simulink model "FINAL_CHB_SPWM_FIXED_DC_5level2"  (R2014a)
settings: Solver=ode45  StartTime=0.0  StopTime=0.4  RelTol=1e-3
libraries: powerlib x22, simulink x4
settings Model: Creator=KOUSIK  LastModifiedBy=PRAKASH BABU

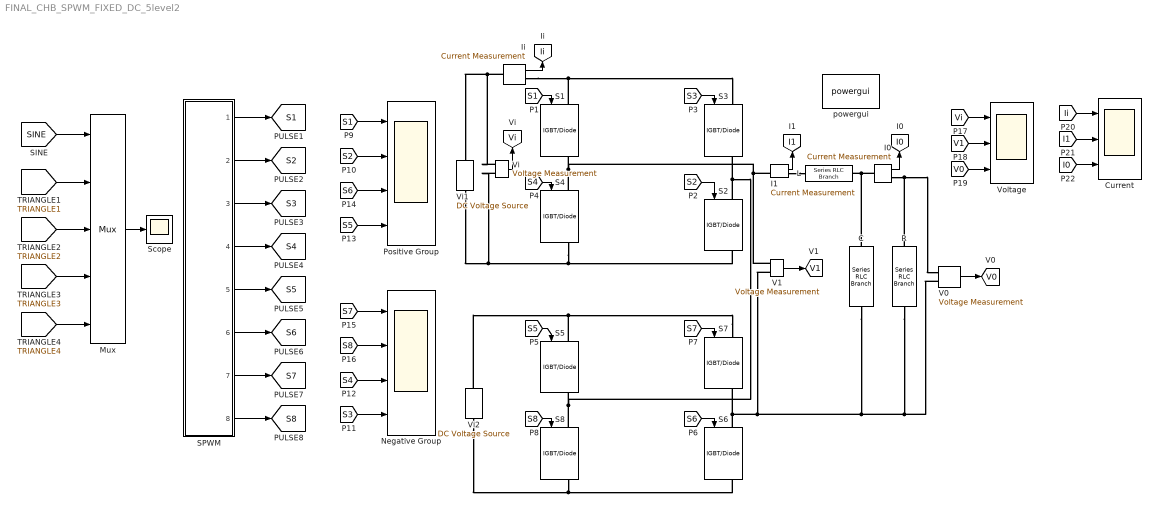
== system FINAL_CHB_SPWM_FIXED_DC_5level2 ==
  C : powerlib/Elements/Series RLC Branch  LConnTagsString=__new0  RConnTagsString=__new0  BranchType=C  Resistance=20  Inductance=5e-3  SetiL0=off  InitialCurrent=0  Capacitance=5.5e-6  Setx0=off  InitialVoltage=0  Measurements=None
  Current : Scope  NumInputPorts=3
      settings: TimeRange=0.1  YMin=-4~-4~-4  YMax=4~4~4  SaveName=current
  I0 : powerlib/Measurements/Current Measurement  PhasorSimulation=off  OutputType=Complex  PSBequivalent=0
  I1 : powerlib/Measurements/Current Measurement  PhasorSimulation=off  OutputType=Complex  PSBequivalent=0
  Ii : powerlib/Measurements/Current Measurement  PhasorSimulation=off  OutputType=Complex  PSBequivalent=0
  L : powerlib/Elements/Series RLC Branch  LConnTagsString=__new0  RConnTagsString=__new0  BranchType=L  Resistance=20  Inductance=35e-3  SetiL0=off  InitialCurrent=0  Capacitance=1e-6  Setx0=off  InitialVoltage=0  Measurements=None
  Mux : Mux  Inputs=5
  Negative Group : Scope  NumInputPorts=4
      settings: YMin=-5~-5~-5~-5  YMax=5~5~5~5  SaveName=negative
  Positive Group : Scope  NumInputPorts=4
      settings: YMin=-5~-5~-5~-5  YMax=5~5~5~5  SaveName=positive
  R : powerlib/Elements/Series RLC Branch  LConnTagsString=__new0  RConnTagsString=__new0  BranchType=R  Resistance=80  Inductance=5e-3  SetiL0=off  InitialCurrent=0  Capacitance=1e-6  Setx0=off  InitialVoltage=0  Measurements=None
  S{1..8} (8 alike) : powerlib/Power Electronics/IGBT//Diode  Ron=1e-3  Rs=1e5  Cs=inf  Measurements=on
  SPWM : Subsystem
  Scope : Scope
      settings: SaveName=sine
  V0 : powerlib/Measurements/Voltage Measurement  PhasorSimulation=off  OutputType=Complex  PSBequivalent=0
  "V1  " : powerlib/Measurements/Voltage Measurement  PhasorSimulation=off  OutputType=Complex  PSBequivalent=0
  Vi : powerlib/Measurements/Voltage Measurement  PhasorSimulation=off  OutputType=Complex  PSBequivalent=0
  Vi1 : powerlib/Electrical Sources/DC Voltage Source  Amplitude=115  Measurements=None
  Vi2 : powerlib/Electrical Sources/DC Voltage Source  Amplitude=115  Measurements=None
  Voltage : Scope  NumInputPorts=3
      settings: TimeRange=0.1  YMin=109~-300~-200  YMax=111~300~200  SaveName=voltage
  powergui : powerlib/powergui  Priority=1  SimulationMode=Discrete  SolverType=Tustin  SampleTime=50e-6  frequency=60  SPID=off  DisableSnubberDevices=off  DisableRonSwitches=off  DisableVfSwitches=off  SwTol=0  Interpol=off  DisplayEquations=off  Ts=0  methode=off  frequencyindice=0  Pbase=100e6  ErrMax=1e-4  Iterations=50  UnitsV=kV  UnitsW=MW  FunctionMessages=off  echomessages=off  HookPort=off  EnableUseOfTLC=off  x0status=blocks  RestoreLinks=warning  ResistiveCurrentMeasurement=off  Frange=[0:2:500]  Ylog=off  Xlog=on  ShowGrid=off  save=off  variable=ZData  structure=voltage  ZoomFFT=off  StartTime=0.02  cycles=1  DisplayStyle=1  fundamental=50  FreqAxis=off  MaxFrequency=1000  frequencyindicesteady=1  RmsSteady=1  display=off
  tag scope: I0=global, I1=global, Ii=global, S1=global, S2=global, S3=global, S4=global, S5=global, S6=global, S7=global, S8=global, V0=global, V1=global, Vi=global
  wires:
  [SINE] -> Mux/1
  [TRIANGLE1] -> Mux/2
  [TRIANGLE2] -> Mux/3
  [TRIANGLE3] -> Mux/4
  [TRIANGLE4] -> Mux/5
  Mux/1 -> Scope/1
  SPWM/1(1) -> [S1]
  SPWM/2(2) -> [S2]
  SPWM/4(4) -> [S4]
  SPWM/5(5) -> [S5]
  SPWM/6(6) -> [S6]
  SPWM/7(7) -> [S7]
  SPWM/8(8) -> [S8]
  SPWM/3(3) -> [S3]
  [S1] -> S1/1
  [S2] -> S2/1
  [S3] -> S3/1
  [S4] -> S4/1
  [S5] -> S5/1
  [S6] -> S6/1
  [S7] -> S7/1
  [S8] -> S8/1
  [S1] -> Positive Group/1
  [S2] -> Positive Group/2
  [S6] -> Positive Group/3
  [S5] -> Positive Group/4
  [S7] -> Negative Group/1
  [S8] -> Negative Group/2
  [S4] -> Negative Group/3
  [S3] -> Negative Group/4
  "V1  "/1 -> [V1]
  Ii/1 -> [Ii]
  Vi/1 -> [Vi]
  I1/1 -> [I1]
  V0/1 -> [V0]
  I0/1 -> [I0]
  [Vi] -> Voltage/1
  [V1] -> Voltage/2
  [V0] -> Voltage/3
  [Ii] -> Current/1
  [I1] -> Current/2
  [I0] -> Current/3
  connections:
  S1/LConn1 -- Ii/RConn1 -- S3/LConn1
  Vi1/LConn1 -- Vi/LConn2 -- S4/RConn1 -- S2/RConn1
  S4/LConn1 -- "V1  "/LConn1 -- I1/LConn1 -- S1/RConn1
  S7/LConn1 -- S5/LConn1 -- Vi2/RConn1
  Vi2/LConn1 -- S8/RConn1 -- S6/RConn1
  S3/RConn1 -- S2/LConn1 -- S8/LConn1 -- S5/RConn1
  S7/RConn1 -- "V1  "/LConn2 -- V0/LConn2 -- R/RConn1 -- C/RConn1 -- S6/LConn1
  Ii/LConn1 -- Vi1/RConn1 -- Vi/LConn1
  C/LConn1 -- L/LConn1 -- I0/LConn1
  R/LConn1 -- V0/LConn1 -- I0/RConn1
  I1/RConn1 -- L/RConn1

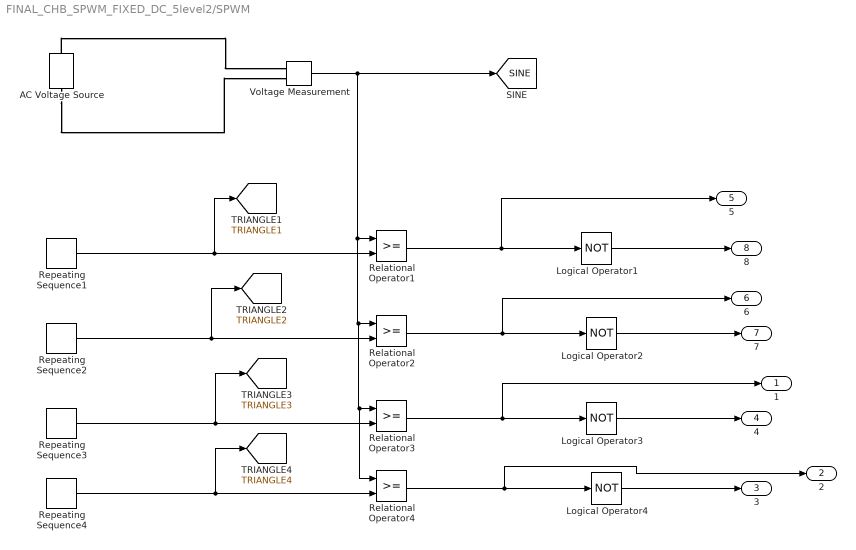
== system FINAL_CHB_SPWM_FIXED_DC_5level2/SPWM ==
  AC Voltage Source : powerlib/Electrical Sources/AC Voltage Source  Amplitude=1.6  Phase=0  Frequency=50  SampleTime=0  Measurements=None
  Logical Operator{1..4} (4 alike) : Logic  Operator=NOT  AllPortsSameDT=off  OutDataTypeStr=boolean
  Relational Operator{1..4} (4 alike) : RelationalOperator  OutDataTypeStr=boolean
  Repeating Sequence1 : simulink/Sources/Repeating Sequence  rep_seq_t=[0 0.5 1]/2500  rep_seq_y=[1 2 1]
  Repeating Sequence2 : simulink/Sources/Repeating Sequence  rep_seq_t=[0 0.5 1]/2500  rep_seq_y=[0 1 0]
  Repeating Sequence3 : simulink/Sources/Repeating Sequence  rep_seq_t=[0 0.5 1]/2500  rep_seq_y=[-1 0 -1]
  Repeating Sequence4 : simulink/Sources/Repeating Sequence  rep_seq_t=[0 0.5 1]/2500  rep_seq_y=[-2 -1 -2]
  Voltage Measurement : powerlib/Measurements/Voltage Measurement  PhasorSimulation=off  OutputType=Complex  PSBequivalent=0
  1 : Outport
  2 : Outport  Port=2
  3 : Outport  Port=3
  4 : Outport  Port=4
  5 : Outport  Port=5
  6 : Outport  Port=6
  7 : Outport  Port=7
  8 : Outport  Port=8
  tag scope: SINE=global, TRIANGLE1=global, TRIANGLE2=global, TRIANGLE3=global, TRIANGLE4=global
  wires:
  Logical Operator1/1 -> 8/1
  Relational Operator1/1 -> 5/1, Logical Operator1/1
  Repeating Sequence2/1 -> [TRIANGLE2], Relational Operator2/2
  Relational Operator2/1 -> 6/1, Logical Operator2/1
  Voltage Measurement/1 -> Relational Operator4/1, Relational Operator3/1, Relational Operator2/1, Relational Operator1/1, [SINE]
  Relational Operator3/1 -> 1/1, Logical Operator3/1
  Repeating Sequence1/1 -> [TRIANGLE1], Relational Operator1/2
  Repeating Sequence3/1 -> [TRIANGLE3], Relational Operator3/2
  Logical Operator2/1 -> 7/1
  Relational Operator4/1 -> 2/1, Logical Operator4/1
  Repeating Sequence4/1 -> [TRIANGLE4], Relational Operator4/2
  Logical Operator3/1 -> 4/1
  Logical Operator4/1 -> 3/1
  connections:
  AC Voltage Source/LConn1 -- Voltage Measurement/LConn2
  AC Voltage Source/RConn1 -- Voltage Measurement/LConn1
